simulink model "TIA"  (R2017b)
settings: Solver=VariableStepAuto  StartTime=0.0  StopTime=inf  RelTol=1e-3
undefined symbols (not defined in the file): sigbuilder_block
(part 2 of 2)

== matlab function TIA/Baler/AutoCfg_1 SubSystem/RearDoorControl/OpenRearDoorFunction ==
  data: StopSignal input; Y output; BaleSize input; RearObstSr input

function Y = fcn(StopSignal,BaleSize,RearObstSr)

if (StopSignal==1 && BaleSize==2 && RearObstSr==0)
    Y =1;
else
    
    Y=0;
    
end

== matlab function TIA/Baler/AutoCfg_1 SubSystem/RearDoorControl/CloseRearDoor ==
  data: DoorStatus input; y output; BaleOutSr input
function y = fcn(DoorStatus, BaleOutSr)
if (DoorStatus==1 &&BaleOutSr==1)
y = 0;
else
 y=DoorStatus;
    
end

== matlab function TIA/Baler/AutoCfg_1 SubSystem/CalcTargetAngel ==
  data: Stop input; SWL input; TargetAngle output
function TargetAngle = fcn(Stop, SWL)
if(Stop==1)
  TargetAngle=0;
else
TargetAngle = 3*SWL;
end

== stateflow chart TIA/Baler/BalerMode1 ==
  state SensorsLogic [parallel]
    settings: executionOrder=1
    state BothSrsWork
      entry: BalerMode=3;
      SysReconfigReq=0;
    state FirstSrFail
      entry:  BalerMode=3.2;
      SysReconfigReq=0;
    state BotheFail
      entry:  BalerMode=1;
      SysReconfigReq=1;
    state SecondSrFail [commented out]
      entry:  BalerMode=2;
      SysReconfigReq=1.2;
    BothSrsWork -> FirstSrFail : [RObstSr_isBroken(RSr1) ]
    (default) -> BothSrsWork
    FirstSrFail -> BothSrsWork [order 2] : [~(RObstSr_isBroken(RSr1))]
    BothSrsWork -> SecondSrFail [commented out] : [RObstSr_isBroken(RSr2)]
    SecondSrFail -> BothSrsWork [commented out] : [~RObstSr_isBroken(RSr2)]
    BotheFail -> BothSrsWork [order 1] : [~(RObstSr_isBroken(RSr1))&&~(RObstSr_isBroken(RSr2))]
    BotheFail -> FirstSrFail [order 2] : [~(RObstSr_isBroken(RSr2))]
    FirstSrFail -> BotheFail [order 1] : [(RObstSr_isBroken(RSr2))]
    SecondSrFail -> BotheFail [commented out] : [RObstSr_isBroken(RSr1)]
    BotheFail -> SecondSrFail [commented out] : [~RObstSr_isBroken(RSr1)]
  state BalerLogic [parallel]
    settings: executionOrder=2
    state Auto
      entry: SysModeOut=3 ;
      ِ
      state Auto3
        entry:BalerCfgMode=3.2;
        AutoCfg_2=true;
        exit:AutoCfg_2=false;
      state Auto1
        entry:BalerCfgMode=3.1;
        AutoCfg_1=true;
        exit:AutoCfg_1=false;
        ِ
      Auto1 -> Auto3 : [ BalerMode==3.2]
      (default) -> Auto1
    state SemiAuto
      entry: SysModeOut=2;
      BalerCfgMode=2;
      SemiAutoCfg=true;
      exit:SemiAutoCfg=false;
    state Manual
      entry: SysModeOut=1;
      BalerCfgMode=1;
      ManualCfg=true;
      exit: ManualCfg=false;
    Manual -> Auto [order 2] : [ModeInput==3]
    Manual -> SemiAuto [order 1] : [ModeInput==2&&(BalerMode~=1)]
    (default) -> Manual
    SemiAuto -> Auto [order 1] : [ModeInput==3]
    SemiAuto -> Manual [order 2] : [ModeInput==1]
    Auto -> SemiAuto [order 3] : [ModeInput==2]
    Auto -> Manual [order 1] : [ModeInput==1]
    Auto -> SemiAuto [order 2] : [( ModeInput==2)]
  data: obst function_input; status function_output; ModeInput input; SysModeOut output; RSr1 input; RSr2 input; BalerCfgMode output; SysReconfigReq output; AutoCfg_1 output; AutoCfg_2 output; SemiAutoCfg output; BalerMode local; ManualCfg output boolean
  function status=RObstSr_isBroken(obst):
    | function status=RObstSr_isBroken(obst)
    |  
    | if ((obst==1)||(obst==0))
    | 
    | status=false;
    | else
    |     status=true;
    | end

== stateflow chart TIA/Tractor/TractorMode ==
  state SystemLogic [parallel]
    settings: executionOrder=1
    state Initial_ReconfigState
      entry: SysModeOut=0;
    state Manual
      entry: SysModeOut=1;
      ManualCfg=true;
      exit:ManualCfg=false;
    state SemiAuto
      entry: SysModeOut=2;
      SemiAutoCfg=true;
      exit:SemiAutoCfg=false;
    state Auto
      entry: SysModeOut=3;
      AutoCfg=true;
      exit:AutoCfg=false;
    (default) -> Initial_ReconfigState
    Initial_ReconfigState -> Auto [order 3] : [ModeInput==3]
    Manual -> Auto [order 2] : [(ModeInput==3)&&(SysReconfigReq~=1)]
    Initial_ReconfigState -> SemiAuto [order 2] : [ModeInput==2]
    Initial_ReconfigState -> Manual [order 1] : [ModeInput==1]
    Auto -> SemiAuto [order 2] : [(ModeInput==2) || (FrontObsSr_isBroken(Fobst))]{ AutoCfg=false;send(Ewarn,UserPresentWarn)}
    Manual -> SemiAuto [order 1] : [ModeInput==2&&((SysReconfigReq~=1)&&(SysReconfigReq~=1.2))]
    SemiAuto -> Manual [order 2] : [(ModeInput==1)||(SysReconfigReq==1)]
    SemiAuto -> Auto [order 1] : [(ModeInput==3)&&(~FrontObsSr_isBroken(Fobst))]
    Auto -> Manual [order 1] : [(ModeInput==1)||(SysReconfigReq==1)]{send(Ewarn,UserPresentWarn)}
  state UserPresentWarn [parallel]
    settings: executionOrder=2
    state Runing
      state OK
      state Stop
      (default) -> OK
      OK -> Stop : [Ewarn]
      Stop -> OK : [UserPresent==1]
    state ShutDown
    (default) -> Runing
    Runing -> ShutDown : [((UserPresent==0)&&((SysModeOut==1)||(SysModeOut==2)))&&after(40,sec)]
    ShutDown -> Runing : [UserPresent==1]
  data: FobstValue function_input; status function_output; ModeInput input; SysModeOut output; Fobst input; AutoCfg output boolean; SemiAutoCfg output boolean; ManualCfg output boolean; SysReconfigReq input; Warn output boolean; UserPresent input; ShutDown output boolean
  events: Ewarn local FUNCTION_CALL_EVENT
  function status = FrontObsSr_isBroken(FobstValue):
    | function status=FrontObsSr_isBroken(FobstValue)
    | 
    | if ((FobstValue==1)||(FobstValue==0))
    | 
    | status=false;
    | else
    |     status=true;
    | end

== stateflow chart TIA/SwathScanner/Chart ==
  state AutoCfg
    state Auto1
      entry: SysModeOut=3.1;
      AutoCfg1=true;
      exit: AutoCfg1=false;
    state Auto2
      entry: SysModeOut=3.2;
      AutoCfg2=true;
      exit:AutoCfg2=false;
    (default) -> (junction 63) [commented out]
    (junction 63) -> Auto2 [commented out] : [isBroken(SpSr1)==true]
    (junction 63) -> Auto1 [commented out] : [[isBroken(SpSr1)==false]]
    Auto1 -> Auto2 : [isBroken(SpSr1)==true]
    (default) -> Auto1
  state SemiAuto
    entry: SysModeOut=2;
    SemiAutoCfg=true;
    exit:SemiAutoCfg=false;
  state Manual
    entry: SysModeOut=1;
    ManualCfg=true;
    exit:ManualCfg=false;
  Manual -> AutoCfg [order 2] : [ModeInput==3]
  AutoCfg -> SemiAuto [order 1] : [ModeInput==2]
  Manual -> SemiAuto [order 1] : [ModeInput==2]
  (default) -> Manual
  SemiAuto -> AutoCfg [order 1] : [ModeInput==3]
  SemiAuto -> Manual [order 2] : [ModeInput==1]
  AutoCfg -> Manual [order 2] : [ModeInput==1]
  data: Speed function_input; status function_output; ModeInput input; SysModeOut output; AutoCfg1 output boolean; AutoCfg2 output boolean; SemiAutoCfg output boolean; SpSr1 input; ManualCfg output boolean
  function status=isBroken(Speed):
    | function status=isBroken(Speed)
    | 
    | if ((Speed>20)||(Speed<0))
    | 
    | status=true;
    | else
    |     status=false;
    | end

== matlab function TIA/SwathScanner/Auto_1_Cfg Subsystem/CalcVolFlowRate 1/MATLAB Function ==
  data: speed input; y output; area input
function y = fcn(speed, area)

y = speed*area;

== matlab function TIA/SwathScanner/Auto_2_Cfg Subsystem/CalcVolFlowRate 1/MATLAB Function ==
  data: speed input; y output; area input
function y = fcn(speed, area)

y = speed*area;

== matlab function TIA/Baler/AutoCfg_2 Subsystem/CalcTargetAngel ==
  data: SWL input; TargetAngle output
function TargetAngle = fcn(SWL)

  
TargetAngle = 3*SWL;
end

== matlab function TIA/Baler/AutoCfg_2 Subsystem/CalcTargetSpeed/MATLAB Function ==
  data: u input; TargetSpeed output
function TargetSpeed = fcn(u)

  
TargetSpeed = -.10*u+20;
end

== matlab function TIA/Baler/AutoCfg_2 Subsystem/RearDoorControl/CloseRearDoor ==
  data: DoorStatus input; y output; BaleOutSr input
function y = fcn(DoorStatus, BaleOutSr)
if (DoorStatus==1 &&BaleOutSr==1)
y = 0;
else
 y=DoorStatus;
    
end

== matlab function TIA/Baler/AutoCfg_2 Subsystem/RearDoorControl/OpenRearDoorFunction ==
  data: StopSignal input; Y output; BaleSize input; RearObstSr input

function Y = fcn(StopSignal,BaleSize,RearObstSr)

if (StopSignal==1 && BaleSize==2 && RearObstSr==0)
    Y =1;
else
    
    Y=0;
    
end

== matlab function TIA/SwathScanner/SemiAuto_Cfg Subsystem/CalcVolFlowRate 1/MATLAB Function ==
  data: speed input; y output; area input
function y = fcn(speed, area)

y = speed*area;

== matlab function TIA/Baler/SemiAutoCfg Subsystem/CalcTargetSpeed/MATLAB Function ==
  data: u input; TargetSpeed output
function TargetSpeed = fcn(u)

  
TargetSpeed = -.10*u+20;
end

== matlab function TIA/Baler/SemiAutoCfg Subsystem/RearDoorControl/CloseRearDoor ==
  data: DoorStatus input; y output; BaleOutSr input
function y = fcn(DoorStatus, BaleOutSr)
if (DoorStatus==1 &&BaleOutSr==1)
y = 0;
else
 y=DoorStatus;
    
end

== matlab function TIA/Baler/SemiAutoCfg Subsystem/RearDoorControl/OpenRearDoorFunction ==
  data: StopSignal input; Y output; BaleSize input; RearObstSr input

function Y = fcn(StopSignal,BaleSize,RearObstSr)

if (StopSignal==1 && BaleSize==2 && RearObstSr==0)
    Y =1;
else
    
    Y=0;
    
end

== matlab function TIA/Tractor/ManualCfg SubSystem/setStAngle ==
  data: TAngle input; CAngle output
function CAngle = fcn( TAngle )


   CAngle = 3*TAngle; 
end

== matlab function TIA/Tractor/Auto_Cfg SubSystem/setStAngle ==
  data: TAngle input; CAngle output
function CAngle = fcn( TAngle )


   CAngle = TAngle; 
end

== matlab function TIA/Tractor/SemiAuto_Cfg SubSystem/setStAngle ==
  data: TAngle input; CAngle output
function CAngle = fcn( TAngle )


   CAngle = 3*TAngle; 
end

== stateflow chart TIA/Tractor/SpeedController ==
  state initial
    entry:Speed=0;
  state Manual
    state Initiate
      entry:Speed=0;
    state accelerate
      du:Speed= Speed +1;
    state Brake
      du:Speed =0;
    state DriveStable
      du:Speed = 4*MTSpeed;
    state decelerate
      du:Speed = Speed - 1;
    (default) -> Manual.Initiate
    Manual.Initiate -> Manual.accelerate : [(Warn==0)&&Shutdown==0]
    Manual.Brake -> Manual.accelerate : [MStopUserInput==0]
    Manual.accelerate -> Manual.DriveStable [order 1] : [Speed==8]
    Manual.accelerate -> Manual.decelerate [order 2] : [MStopUserInput==1]
    Manual.decelerate -> Manual.accelerate [order 1] : [MStopUserInput~=1]
    Manual.decelerate -> Manual.Brake [order 2] : [Speed<=5]
    Manual.DriveStable -> Manual.decelerate : [MStopUserInput==1]
  state Semi
    state Initiate
      entry:Speed=0;
    state accelerate
      du:Speed= Speed +1;
    state DriveStable
      du:Speed = BTSpeed;
    state Brake
      du:Speed =0;
    state SlowDrive
      du:Speed =5;
    state decelerate
      du:Speed = Speed - 1;
    (default) -> Semi.Initiate
    Semi.Initiate -> Semi.accelerate : [(Warn==0)&&(Shutdown==0)]
    Semi.SlowDrive -> Semi.accelerate [order 2] : [BStopUserInput~=1&&(BBaleSize==0)]
    Semi.accelerate -> Semi.DriveStable [order 1] : [Speed==8]
    Semi.Brake -> Semi.accelerate : [BStopUserInput==0&&(BBaleSize==0)]
    Semi.accelerate -> Semi.decelerate [order 2] : [BStopUserInput==1]
    Semi.decelerate -> Semi.accelerate [order 1] : [BStopUserInput~=1&&(BBaleSize==0)]
    Semi.DriveStable -> Semi.decelerate : [BStopUserInput==1||(BBaleSize==1)]
    (junction 139) -> Semi.Brake [order 1] : [(BBaleSize==2)||(BStopUserInput==1)]
    Semi.SlowDrive -> Semi.Brake [order 1] : [(BBaleSize==2)||(BStopUserInput==1)]
    (junction 139) -> Semi.SlowDrive [order 2] : [(BBaleSize~=2)&&(BStopUserInput==0)]
    Semi.decelerate -> (junction 139) [order 2] : [Speed<=5]
  state Auto
    state Initiate
      entry:Speed=0;
      du:Speed = Speed +1;
    state Accelerate
      du:Speed= Speed +1;
    state DriveStable
      du:Speed = ATSpeed;
    state Brake
      du:Speed =0;
    state Decelerate
      du:Speed = Speed - 1;
    state SlowDrive
      du:Speed= 5;
    (default) -> Auto.Initiate
    Auto.SlowDrive -> Accelerate [order 2] : [AFObstSr==0&&ABaleSize==0]
    Auto.Brake -> Accelerate : [AFObstSr==0&&(ABaleSize~=2) &&after(30,sec)]
    Accelerate -> Auto.DriveStable [order 1] : [Speed==8]
    Auto.Initiate -> Auto.DriveStable : [Speed==8]
    Accelerate -> Decelerate [order 2] : [AFObstSr==1]
    Decelerate -> Accelerate [order 1] : [AFObstSr~=1&&(ABaleSize==0)]
    Auto.DriveStable -> Decelerate : [AFObstSr==1||(ABaleSize==1)]
    (junction 143) -> Auto.Brake [order 2] : [((AObstDist<=2.5)&&(AFObstSr==1))||(ABaleSize==2)]
    Auto.SlowDrive -> Auto.Brake [order 1] : [(AObstDist<=2.5)||(ABaleSize==2)]
    Decelerate -> (junction 143) [order 2] : [Speed<8]
    (junction 143) -> Auto.SlowDrive [order 1] : [AObstDist>2.5 &&ABaleSize~=2]
  state ReConfigDecelerate
    du:Speed=Speed-1;
  (default) -> initial
  initial -> Auto [order 1] : [SysMode==3]
  initial -> Semi [order 2] : [SysMode==2]
  initial -> Manual [order 3] : [SysMode==1]
  Semi -> ReConfigDecelerate [order 2] : [SysMode==3]
  Semi -> ReConfigDecelerate [order 1] : [SysMode==1]
  ReConfigDecelerate -> Semi [order 2] : [Speed<=3&&(SysMode==2)]
  ReConfigDecelerate -> Manual [order 1] : [Speed<=3&&(SysMode==1)]
  Manual -> ReConfigDecelerate [order 1] : [SysMode==3]
  Manual -> ReConfigDecelerate [order 2] : [SysMode==2]
  Auto -> ReConfigDecelerate [order 1] : [SysMode==1]
  ReConfigDecelerate -> Auto [order 3] : [(Speed<=3)&&(SysMode==3)]
  Auto -> ReConfigDecelerate [order 2] : [SysMode==2]
  data: SysMode input; ACSpeed input; ATSpeed input; ABaleSize input; AFObstSr input; AObstDist input; BCSpeed input; BTSpeed input; BBaleSize input; BStopUserInput input; MCSpeed input; MTSpeed input; MStopUserInput input; Warn input; Speed output; Shutdown input
